simulink model "AUAV_V3_TestSensors"  (R2015a)
settings: Solver=FixedStepDiscrete  StartTime=0.0  StopTime=10.0  FixedStep=T  RelTol=1e-3
PreLoadFcn:
  | %T = 0.0025;
  | MavlinkBus;
  | mcuInit;
  | % Baro Altitude Computation
  | % =========================
  | basePressure = 98192.64;
  | baseTemp = 288.215;
  | lapseRate = -0.00198122;
  | baseHeight = 0;
undefined symbols (not defined in the file): A0, A14, A15, A2, A3, A4, A5, A6, accBiasRateLimit, apSampleTime, B0, bankCommandLimit, barAdjust, baroCutoff, baroCutTemp, baroOffset, baroScale, barTGain1, barTGain2, barTMean1, barTMean2, bda, bde, bdr, bdt, bICda, bICde, bICdr, bICdt, cubeAccelGain16405, cubeGyroGain16405, cubeMagGain16405, D0, D11, D7, D8, daLimit, data, daTrimMax, daTrimMin, deLimit, derivativesConstant, deTrimMax, deTrimMin, drLimit, drTrimMax, drTrimMin, dtLimit, dtTrimMax, dtTrimMin, F2, F3, G0, G13, G15, gaind, GS_location, gyroBiasRateLimit, IC1max, imuOffset_xacc ... (+77)
libraries: MCHP_Blockset x158, simulink x84, SLUGS_Library x31, aerolibconvert2 x6, aerolibutil x4, aerolibtransform2 x3, dspmtrx3 x2, aerolibobsolete x2
(part 8 of 23)

== system AUAV_V3_TestSensors/Trim Vals [updated 4.28.16] ==
  Bufffer IC : Subsystem
  Control Surfaces [dT dA dR dE] : Selector  InputPortWidth=5  Indices=[3 1 4 2]
  Control Surface Input : Subsystem
  "Convert to Microseconds " : Subsystem
  Detect Transition High to Low : Subsystem
  Failsafe : Selector  InputPortWidth=5  Indices=[5]
  Grab I.C. : Subsystem  TreatAsAtomicUnit=on
  Manual or Auto? [navSupport.c] [updated 4.28.16] : MCHP_Blockset/User Functions/C Function Call  ParseFilesChkbx=off  ListFunctions1=Custom Function  Function1=extern uint8_T isApManual(uint16_T u1);  AddHeaderDeclaration=on  Function1Type=when block is updated (default)  FctReturnBlockOut=on  Fct1BlockOut=y1  DataCollected=0  ORDERING=None  SampleTime=-1  MCHP_MASTERLINK=|  PinDigitalInput=[]  PinDigitalOutput=[]  PinAnalogInput=[]
      | AUAV_V3_TestSensors/Microchip Master
      | AUAV V3 Board
      | Busy Flag on D2 (RA6)
  Mean Filter the Transition : Subsystem
  dT Trim : Outport
  dA Trim : Outport  Port=2
  dR Trim : Outport  Port=3
  dE Trim : Outport  Port=4
  Pil Console : Outport  Port=5
  Manual? : Outport  Port=6
  V/I Sensor : Outport  Port=7
  wires:
  Manual or Auto? [navSupport.c] [updated 4.28.16]/1 -> Detect Transition High to Low/1(Switch), Manual?/1
  Control Surface Input/1(Pilot Console) -> Control Surfaces [dT dA dR dE]/1, Failsafe/1
  Control Surfaces [dT dA dR dE]/1 -> Pil Console/1, Bufffer IC/1(Pilot Console)
  Bufffer IC/1(dT_buf) -> Grab I.C./1(dT_buf)
  Bufffer IC/2(dA_buf) -> Grab I.C./2(dA_buf)
  Bufffer IC/3(dR_buf) -> Grab I.C./3(dR_buf)
  Bufffer IC/4(dE_buf) -> Grab I.C./4(dE_buf)
  Grab I.C./4(dE_trim (rad)) -> dE Trim/1
  Grab I.C./3(dR_trim (rad)) -> dR Trim/1
  Grab I.C./2(dA_trim (rad)) -> dA Trim/1
  Grab I.C./1(dT_trim (abs)) -> dT Trim/1
  Detect Transition High to Low/1(Transition) -> Grab I.C./Enable
  Failsafe/1 -> "Convert to Microseconds "/1(IC)
  "Convert to Microseconds "/1(uS) -> Mean Filter the Transition/1(Failsafe)
  Control Surface Input/2(Voltage/Current Sensor) -> V/I Sensor/1
  Mean Filter the Transition/1(filtered) -> Manual or Auto? [navSupport.c] [updated 4.28.16]/1

== system AUAV_V3_TestSensors/Update PWM Commands and Send Telemetry [updated 4.27.16] ==
  PWM(rad) [dT dA dR dE] : Inport
  Pilot Console (IC) [dT dA dR dE] : Inport  Port=2
  Euler_rot : Inport  Port=3
  PQR_rot : Inport  Port=4
  Manual? : Inport  Port=5
  VI : Inport  Port=6
  Convert to Microseconds : Subsystem
  Data Store Read : DataStoreRead  DialogController=Simulink.DDGSource  DataStoreName=SIX_DOF_HIL_FLAG
  Data Store Read1 : DataStoreRead  DataStoreName=X_PLANE_HIL_FLAG
  Demux : Demux
  Demux1 : Demux
  Demux2 : Demux  Outputs=3
  Demux3 : Demux  Outputs=3
  Demux4 : Demux  Outputs=2
  Gain : Gain  Gain=2  OutDataTypeStr=Inherit: Inherit via back propagation
  Generate PWM Signals Based on the Control Type : Subsystem
  Get time3 : DataStoreRead  DataStoreName=time_since_boot_usec  DataStoreElements=time_since_boot_usec
  Output Compare - HW Drive Servo motor : MCHP_Blockset/Pulse Input//Output/Output Compare - HW  Channel="[1     2     3     4]"  Channel_OLD="[1     2     3     4]"  PIN_OC1=Dynamic Options  PIN_OC1_TXT=G0 / P112 / Pin[90]  PIN_OC2=Dynamic Options  PIN_OC2_TXT=E0 / P80 / Pin[93]  PIN_OC3=Dynamic Options  PIN_OC3_TXT=G13 / P125 / Pin[97]  PIN_OC4=Dynamic Options  PIN_OC4_TXT=D7 / P71 / Pin[84]  PIN_OC5=Dynamic Options  PIN_OC5_TXT=D0 / P64 / Pin[72]  PIN_OC6=Dynamic Options  PIN_OC6_TXT=D0 / P64 / Pin[72]  PIN_OC7=Dynamic Options  PIN_OC7_TXT=D0 / P64 / Pin[72]  PIN_OC8=Dynamic Options  PIN_OC8_TXT=D0 / P64 / Pin[72]  PIN_OC9=Dynamic Options  PIN_OC9_TXT=D0 / P64 / Pin[72]  PIN_OC10=Dynamic Options  PIN_OC10_TXT=D0 / P64 / Pin[72]  PIN_OC11=Dynamic Options  PIN_OC11_TXT=D0 / P64 / Pin[72]  PIN_OC12=Dynamic Options  PIN_OC12_TXT=D0 / P64 / Pin[72]  PIN_OC13=Dynamic Options  PIN_OC13_TXT=D0 / P64 / Pin[72]  PIN_OC14=Dynamic Options  PIN_OC14_TXT=D0 / P64 / Pin[72]  PIN_OC15=Dynamic Options  PIN_OC15_TXT=D0 / P64 / Pin[72]  PIN_OC16=Dynamic Options  PIN_OC16_TXT=D0 / P64 / Pin[72]  PIN_OCFA=Dynamic Options  PIN_OCFA_TXT=A0 / P16 / Pin[17]  PIN_OCFB=Dynamic Options  PIN_OCFB_TXT=A0 / P16 / Pin[17]  PIN_OCFC=Dynamic Options  PIN_OCFC_TXT=A0 / P16 / Pin[17]  Channel_UP_Down_Periode="[5     5     5     5]"  PulseTrig=Single pulse triggered by block execution  InputPeriod=are set to the Max time (constant below)  MaxChannel="[0.003   0.003   0.003   0.003]"  MaxChannelUnique=.0001  MaxChannelValue="2.^[ 14.680  14.680  14.680  14.680]  =>  [26249  26249  26249  26249]"  OCxmax="[26249  26249  26249  26249]"  Timer="[1  1  1  1]"  SampleTime=0.02  MCHP_PORT={Output Compare 1}{OC1}7:1:P112;{Output Compare 2}{OC2}7:1:P80;{Output Compare 3}{OC3}7:1:P125;{Output Compare 4}{OC4}7:1:P71;  MCHP_TIMER_REQUEST="{Output Compare 1}{OC1}7:0:1:0:[1  2  3  4  5]:210000;{Output Compare 1}{OC1}7:0:1:0:[1  2  3  4  5]:210000;{Output Compare 1}{OC1}7:0:1:0:[1  2  3  4  5]:210000;{Output Compare 1}{OC1}7:0:1:0:[1  2  3  4  5]:210000;"  MCHP_TIMER_RESULT=[1 26249.000000000011 ;1 26249.000000000011 ;1 26249.000000000011 ;1 26249.000000000011 ]  MCHP_MASTERLINK=|
      | AUAV_V3_TestSensors/Microchip Master
      | AUAV V3 Board
      | Busy Flag on D2 (RA6)
  PWM High Speed : MCHP_Blockset/PWM IO/PWM High Speed  Commented=on  pop1=[1]  chk1="[1  1  1  0]"  chkHL1="[1  1  1  1  0  0  1 ; 1  1  1  1  0  0  1]"  maxP1="[0.001       0.001       0.001       0.001       0.001       0.001       0.001 ; 0.001       0.001      1e-006       0.001       0.001       0.001       0.001]"  InitP2="[0.001       0.001       0.001       0.001       0.001       0.001       0.001 ; 0.001       0.001       0.001       0.001       0.001       0.001       0.001]"  chkP2="[0  0  0  0  1  1  1 ; 1  0  0  1  1  1  1]"  InitDC="[0.0005       0.0004       0.0003        0.001        0.001        0.001           50 ; 0.001        0.001        0.001        0.001        0.001        0.001           50]"  chkDC="[1  1  1  1  1  1  1 ; 0  0  0  1  1  1  1]"  InitPh="[0           0           0       0.001       0.001       0.001       0.001 ; 0           0           0       0.001       0.001       0.001       0.001]"  chkPh="[0  0  0  1  1  1  1 ; 0  0  0  1  1  1  1]"  edSEvTrigx={'0.0006','-1','-1','-1','-1','-1','-1'}  chkSEvTrigx="[0  0  0  0  1  1  1]"  popFlt="[1  1  1  1  1  1  1]"  popFltPin="[48  48  48  48  48  48  48]"  popFltPinRp="[1  1  1  1  1  1  1]"  popFltActivH="[1  2  1  1  1  1  1]"  popFltForceH="[2  2  2  2  2  2  2]"  popFltForceL="[1  1  1  1  1  1  1]"  chkFltBlkOut="[0  0  0  0  0  0  0]"  popDT="[3  3  3  3  3  3  3]"  edDTRx="[0.02      1e-005       0.001      1e-005      1e-005      1e-005      1e-005]"  edAltDTRx="[1e-005      0.0001      1e-005      1e-005      1e-005      1e-005      1e-005]"  S_INPUT="[5  5  5  5]"  S_INPUT_Size=[1 1 1 1]  S_OUTPUT=[]  S_OUTPUT_Size=[]  S_DWORK_Type=[]  S_DWORK_Size=[]  ADC_VARTRIG={PWM Primary Special Event Trigger;6}  SampleTime=-1  ORDERING=None  MCHP_PORT={PWM1H}{PWM1H}4:4:E1;{PWM1L}{PWM1L}4:4:E0;{PWM2H}{PWM2H}4:4:E3;{PWM2L}{PWM2L}4:4:E2;{PWM3H}{PWM3H}4:4:E5;{PWM3L}{PWM3L}4:4:E4;{PWM4H}{PWM4H}4:4:E7;{PWM4L}{PWM4L}4:4:E6;  MCHP_MASTERLINK=|  MCHP_VERSION=v3.38
      | AUAV_V3_TestSensors/Microchip Master
      | AUAV V3 Board
      | Busy Flag on D2 (RA6)
  Rate Transition : RateTransition
  Send_Cmd_6DOF_HIL : Subsystem
  Send_Cmd_X_Plane_HIL : Subsystem
  "[ dA dE dT dR ]" : Selector  InputPortWidth=4  Indices=[2 4 1 3]
  mlAttitude : DataStoreWrite  DataStoreName=mlVISensor  DataStoreElements=mlVISensor.voltage#mlVISensor.reading2
  mlAttitudeEuler : DataStoreWrite  DialogController=Simulink.DDGSource  DataStoreName=mlAttitudeSol  DataStoreElements=mlAttitudeSol.roll#mlAttitudeSol.pitch#mlAttitudeSol.yaw#mlAttitudeSol.time_boot_ms
  mlAttitudePQR : DataStoreWrite  DialogController=Simulink.DDGSource  DataStoreName=mlAttitudeSol  DataStoreElements=mlAttitudeSol.rollspeed#mlAttitudeSol.pitchspeed#mlAttitudeSol.yawspeed
  mlHeartbeatLocal : DataStoreRead  DataStoreName=mlHeartbeatLocal  DataStoreElements=mlHeartbeatLocal.custom_mode
  mlPwmCommands : DataStoreWrite  DialogController=Simulink.DDGSource  DataStoreName=mlPwmCommands  DataStoreElements=mlPwmCommands.servo1_raw#mlPwmCommands.servo2_raw#mlPwmCommands.servo3_raw#mlPwmCommands.servo4_raw#mlPwmCommands.time_usec
  wires:
  Generate PWM Signals Based on the Control Type/1(PWM) -> "[ dA dE dT dR ]"/1, Convert to Microseconds/1(PWM)  "[dT dA dR dE]"
  PWM(rad) [dT dA dR dE]/1 -> Generate PWM Signals Based on the Control Type/1(PWM(rad))
  Pilot Console (IC) [dT dA dR dE]/1 -> Generate PWM Signals Based on the Control Type/2(Pilot Console (IC))
  Manual?/1 -> Generate PWM Signals Based on the Control Type/3(isManual?)
  mlHeartbeatLocal/1 -> Generate PWM Signals Based on the Control Type/4(Nav Mode)
  Convert to Microseconds/1(uS) -> Demux1/1
  Demux1/1 -> mlPwmCommands/1
  Demux1/2 -> mlPwmCommands/2
  Demux1/3 -> mlPwmCommands/3
  Demux1/4 -> mlPwmCommands/4
  Demux2/1 -> mlAttitudeEuler/1
  Demux2/2 -> mlAttitudeEuler/2
  Demux2/3 -> mlAttitudeEuler/3
  Euler_rot/1 -> Demux2/1
  Demux3/1 -> mlAttitudePQR/1
  Demux3/2 -> mlAttitudePQR/2
  Demux3/3 -> mlAttitudePQR/3
  PQR_rot/1 -> Demux3/1
  Demux4/1 -> mlAttitude/1
  Demux4/2 -> mlAttitude/2
  VI/1 -> Demux4/1
  Demux/1 -> Output Compare - HW Drive Servo motor/1
  Demux/2 -> Output Compare - HW Drive Servo motor/2
  Demux/3 -> Output Compare - HW Drive Servo motor/3
  Demux/4 -> Output Compare - HW Drive Servo motor/4
  Get time3/1 -> mlPwmCommands/5, mlAttitudeEuler/4
  Data Store Read/1 -> Send_Cmd_6DOF_HIL/Enable
  Data Store Read1/1 -> Send_Cmd_X_Plane_HIL/Enable
  "[ dA dE dT dR ]"/1 -> Rate Transition/1
  Rate Transition/1 -> Gain/1
  Gain/1 -> Demux/1

== system AUAV_V3_TestSensors/get Nav Vars [updated 4.28.16] ==
  Attitude : Inport
  Accel : Inport  Port=2
  Accel. Bias : Inport  Port=3
  Angle Conversion : aerolibconvert2/Angle Conversion  IU=deg  OU=rad
  Demux : Demux  Outputs=3
  Direction Cosine Matrix to Rotation Angles : aerolibtransform2/Direction Cosine Matrix to Rotation Angles  rotationOrder=ZYX  lim=Default
      settings: AttributesFormatString=Rotation Order: %<rotationOrder>
  Embedded MATLAB Function1 : MATLAB Function  TreatAsAtomicUnit=on
  Euler : Selector  InputPortWidth=6  Indices=[1 2 3]
  Euler Angles to Direction Cosine Matrix1 : aerolibobsolete/Euler Angles to  Direction Cosine Matrix
  Euler Angles to Direction Cosine Matrix2 : aerolibobsolete/Euler Angles to  Direction Cosine Matrix
  Math Function : Math  Operator=transpose  SaturateOnIntegerOverflow=on
  Mux : Mux  Inputs=3
  PAR_CONFIG_ROLL_R PAR_CONFIG_PITCH_R PAR_CONFIG_YAW_R : DataStoreRead  DialogController=Simulink.DDGSource  DataStoreName=mlParamInterface  DataStoreElements=mlParamInterface.param(16)#mlParamInterface.param(17)#mlParamInterface.param(18)
  Product{,1..3} (4 alike) : Product  Multiplication=Matrix(*)  RndMeth=Zero
  Rates : Selector  InputPortWidth=6  Indices=[4 5 6]
  Selector : Selector  InputPortWidth=6  Indices=[1 2 5 6]
  Selector1 : Selector  InputPortWidth=3  Indices=[2]
  Sum : Sum  Inputs=+|+
  myMux Fun1 : MATLAB Function  TreatAsAtomicUnit=on
  myMux Fun2 : MATLAB Function  TreatAsAtomicUnit=on
  "[phi the q r]" : Outport
  Euler Rot : Outport  Port=2
  PQR Rot : Outport  Port=3
  Yb Accel : Outport  Port=4
  wires:
  Selector/1 -> "[phi the q r]"/1
  Euler/1 -> Euler Angles to Direction Cosine Matrix2/1
  Euler Angles to Direction Cosine Matrix2/1 -> Product/2
  Euler Angles to Direction Cosine Matrix1/1 -> Math Function/1
  Angle Conversion/1 -> Euler Angles to Direction Cosine Matrix1/1
  Product/1 -> Direction Cosine Matrix to Rotation Angles/1
  Rates/1 -> Product1/2
  myMux Fun1/1(y) -> Euler Rot/1, myMux Fun2/1(u1)
  Product1/1 -> myMux Fun2/2(u2), PQR Rot/1
  myMux Fun2/1(y) -> Selector/1
  Math Function/1 -> Product/1, Product1/1, Product2/1, Product3/1
  Accel/1 -> Product2/2
  Accel. Bias/1 -> Product3/2
  Product2/1 -> Sum/1
  Product3/1 -> Sum/2
  Sum/1 -> Selector1/1
  Selector1/1 -> Yb Accel/1
  Demux/1 -> Embedded MATLAB Function1/1(u)
  Direction Cosine Matrix to Rotation Angles/1 -> Demux/1
  Demux/2 -> myMux Fun1/2(u2)
  Demux/3 -> myMux Fun1/1(u1)
  Embedded MATLAB Function1/1(y) -> myMux Fun1/3(u3)
  Attitude/1 -> Euler/1, Rates/1
  PAR_CONFIG_ROLL_R PAR_CONFIG_PITCH_R PAR_CONFIG_YAW_R/2 -> Mux/2
  PAR_CONFIG_ROLL_R PAR_CONFIG_PITCH_R PAR_CONFIG_YAW_R/1 -> Mux/1
  PAR_CONFIG_ROLL_R PAR_CONFIG_PITCH_R PAR_CONFIG_YAW_R/3 -> Mux/3
  Mux/1 -> Angle Conversion/1

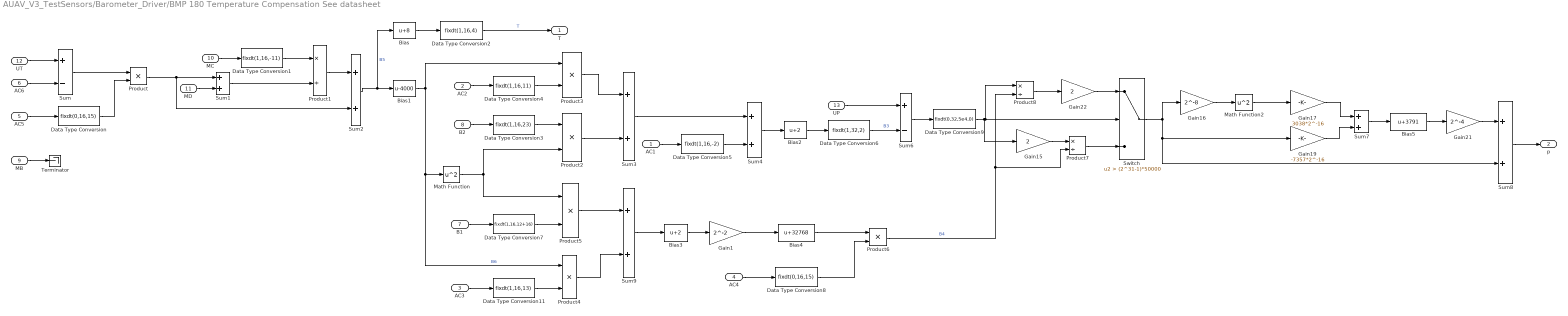
== system AUAV_V3_TestSensors/Barometer_Driver/BMP 180 Temperature Compensation See datasheet ==
  AC1 : Inport
  AC2 : Inport  Port=2
  AC3 : Inport  Port=3
  AC4 : Inport  Port=4
  AC5 : Inport  Port=5
  AC6 : Inport  Port=6
  B1 : Inport  Port=7
  B2 : Inport  Port=8
  MB : Inport  Port=9
  MC : Inport  Port=10
  MD : Inport  Port=11
  UT : Inport  Port=12
  UP : Inport  Port=13
  Bias : Bias  Bias=8
  Bias1 : Bias  Bias=-4000
  Bias2 : Bias  Bias=2
  Bias3 : Bias  Bias=2
  Bias4 : Bias  Bias=32768
  Bias5 : Bias  Bias=3791
  Data Type Conversion : DataTypeConversion  OutDataTypeStr=fixdt(0,16,15)  ConvertRealWorld=Stored Integer (SI)
  Data Type Conversion1 : DataTypeConversion  OutDataTypeStr=fixdt(1,16,-11)  ConvertRealWorld=Stored Integer (SI)
  Data Type Conversion11 : DataTypeConversion  OutDataTypeStr=fixdt(1,16,13)  ConvertRealWorld=Stored Integer (SI)
  Data Type Conversion2 : DataTypeConversion  OutDataTypeStr=fixdt(1,16,4)  ConvertRealWorld=Stored Integer (SI)
  Data Type Conversion3 : DataTypeConversion  OutDataTypeStr=fixdt(1,16,23)  ConvertRealWorld=Stored Integer (SI)
  Data Type Conversion4 : DataTypeConversion  OutDataTypeStr=fixdt(1,16,11)  ConvertRealWorld=Stored Integer (SI)
  Data Type Conversion5 : DataTypeConversion  OutDataTypeStr=fixdt(1,16,-2)  ConvertRealWorld=Stored Integer (SI)
  Data Type Conversion6 : DataTypeConversion  OutDataTypeStr=fixdt(1,32,2)  ConvertRealWorld=Stored Integer (SI)
  Data Type Conversion7 : DataTypeConversion  OutDataTypeStr=fixdt(1,16,12+16)  ConvertRealWorld=Stored Integer (SI)
  Data Type Conversion8 : DataTypeConversion  OutDataTypeStr=fixdt(0,16,15)  ConvertRealWorld=Stored Integer (SI)
  Data Type Conversion9 : DataTypeConversion  OutDataTypeStr=fixdt(0,32,5e4,0)  ConvertRealWorld=Stored Integer (SI)
  Gain1 : Gain  Gain=2^-2  OutDataTypeStr=int32
  Gain15 : Gain  Gain=2  OutDataTypeStr=uint32  RndMeth=Round
  Gain16 : Gain  Gain=2^-8  OutDataTypeStr=int32  RndMeth=Round
  Gain17 : Gain  Gain=3038*2^-16  OutDataTypeStr=uint32
  Gain19 : Gain  Gain=-7357*2^-16  ParamDataTypeStr=fixdt(1,16)  OutDataTypeStr=int32
  Gain21 : Gain  Gain=2^-4  OutDataTypeStr=Inherit: Same as input
  Gain22 : Gain  Gain=2  OutDataTypeStr=Inherit: Same as input
  Math Function : Math  Operator=square  SaturateOnIntegerOverflow=on  OutDataTypeStr=Inherit: Inherit via internal rule
  Math Function2 : Math  Operator=square  OutDataTypeStr=uint32  SaturateOnIntegerOverflow=on
  Product : Product  RndMeth=Round  OutDataTypeStr=Inherit: Same as first input
  Product1 : Product  Inputs=*/  OutDataTypeStr=int16  RndMeth=Round
  Product2 : Product  OutDataTypeStr=int16
  Product3 : Product  OutDataTypeStr=Inherit: Same as first input
  Product4 : Product  OutDataTypeStr=int16
  Product5 : Product  OutDataTypeStr=int16
  Product6 : Product  OutDataTypeStr=uint32
  Product7 : Product  Inputs=*/  RndMeth=Round
  Product8 : Product  Inputs=*/  OutDataTypeStr=uint32  RndMeth=Round
  Sum : Sum  Inputs=+-  RndMeth=Round
  Sum1 : Sum  RndMeth=Round  OutDataTypeStr=Inherit: Same as first input
  Sum2 : Sum  AccumDataTypeStr=int16  OutDataTypeStr=int16  RndMeth=Round
  Sum3 : Sum
  Sum4 : Sum  OutDataTypeStr=int32
  Sum6 : Sum  Inputs=+-  AccumDataTypeStr=uint32  OutDataTypeStr=uint32
  Sum7 : Sum  AccumDataTypeStr=int32  OutDataTypeStr=int32
  Sum8 : Sum  AccumDataTypeStr=int32  OutDataTypeStr=Inherit: Same as accumulator  RndMeth=Round
  Sum9 : Sum
  Switch : Switch  Criteria=u2 > Threshold  Threshold=(2^31-1)*50000
  Terminator : Terminator
  T : Outport
  p : Outport  Port=2
  wires:
  MB/1 -> Terminator/1
  Sum9/1 -> Bias3/1
  Product4/1 -> Sum9/2
  Product5/1 -> Sum9/1
  Product2/1 -> Sum3/2
  Product3/1 -> Sum3/1
  Data Type Conversion3/1 -> Product2/1
  Data Type Conversion11/1 -> Product4/2
  Product1/1 -> Sum2/1
  Data Type Conversion8/1 -> Product6/2
  Data Type Conversion7/1 -> Product5/2
  Data Type Conversion4/1 -> Product3/2
  Math Function/1 -> Product5/1, Product2/2
  Data Type Conversion/1 -> Product/2
  Bias5/1 -> Gain21/1
  Sum8/1 -> p/1
  Gain21/1 -> Sum8/1
  Sum7/1 -> Bias5/1
  Gain17/1 -> Sum7/1
  Gain19/1 -> Sum7/2
  Math Function2/1 -> Gain17/1
  Gain16/1 -> Math Function2/1
  Switch/1 -> Gain19/1, Sum8/2, Gain16/1
  Product7/1 -> Switch/3
  Product8/1 -> Gain22/1
  Data Type Conversion9/1 -> Gain15/1, Product8/1, Switch/2
  Sum6/1 -> Data Type Conversion9/1
  UP/1 -> Sum6/1
  Data Type Conversion6/1 -> Sum6/2  "B3"
  Product6/1 -> Product8/2, Product7/2  "B4"
  Bias4/1 -> Product6/1
  AC4/1 -> Data Type Conversion8/1
  Gain1/1 -> Bias4/1
  Bias3/1 -> Gain1/1
  B1/1 -> Data Type Conversion7/1
  AC3/1 -> Data Type Conversion11/1
  Sum4/1 -> Bias2/1
  Data Type Conversion5/1 -> Sum4/2
  Bias2/1 -> Data Type Conversion6/1
  AC1/1 -> Data Type Conversion5/1
  Sum3/1 -> Sum4/1
  AC2/1 -> Data Type Conversion4/1
  B2/1 -> Data Type Conversion3/1
  Bias1/1 -> Product3/1, Product4/1, Math Function/1  "B6"
  MC/1 -> Data Type Conversion1/1
  Data Type Conversion2/1 -> T/1  "T"
  Bias/1 -> Data Type Conversion2/1
  Sum1/1 -> Product1/2
  Sum2/1 -> Bias1/1, Bias/1  "B5"
  Product/1 -> Sum1/1, Sum2/2
  MD/1 -> Sum1/2
  AC5/1 -> Data Type Conversion/1
  Sum/1 -> Product/1
  AC6/1 -> Sum/2
  UT/1 -> Sum/1
  Data Type Conversion1/1 -> Product1/1
  Gain22/1 -> Switch/1
  Gain15/1 -> Product7/1

== system AUAV_V3_TestSensors/Barometer_Driver/Baro Altimeter ==
  Static (Pa) : Inport
  Compute Barometric Height : Subsystem  mask{baseTemp=baseTemp, LapseRate=lapseRate}
      mask prompts: baseTemp "Base Station Temperature (K)"; LapseRate "Lapse Rate (C/ft)"
      mask help:
      | Produces Altitude in meters from Barometric Pressure in Pascals. Altitude is valid from MSL to 6000 ft.
      |
      | The method implemented here was developed by Ren Curry
  Constant5 : Constant  Value=baseHeight  OutDataTypeStr=single
  Enabled Subsystem : Subsystem  TreatAsAtomicUnit=on
  Enables/Disables the Computation of initial Baro Bias : MATLAB Function  TreatAsAtomicUnit=on
  Initial Baro Bias : Subsystem  TreatAsAtomicUnit=on
  Logical Operator : Logic  Operator=NOT  AllPortsSameDT=off  OutDataTypeStr=boolean
  Sum1 : Sum  Inputs=++|  OutDataTypeStr=single
  Zero Out Height : Subsystem  TreatAsAtomicUnit=on
  Altitude : Outport
  wires:
  Enabled Subsystem/1(Out1) -> Altitude/1
  Sum1/1 -> Enabled Subsystem/1(In1)
  Logical Operator/1 -> Enabled Subsystem/Enable
  Zero Out Height/1(Height Offset) -> Sum1/1
  Initial Baro Bias/1(Baro (Gnd)) -> Compute Barometric Height/2(Base Pressure (Pa))
  Constant5/1 -> Zero Out Height/1(Base Height), Compute Barometric Height/1(Base Height (m))
  Enables/Disables the Computation of initial Baro Bias/1(tOut) -> Logical Operator/1, Zero Out Height/Enable, Initial Baro Bias/Enable
  Static (Pa)/1 -> Compute Barometric Height/3(Baro (Pa)), Initial Baro Bias/1(Baro (Pa))
  Compute Barometric Height/1("Altitude, m") -> Sum1/2, Zero Out Height/2(Computed Height)

== system AUAV_V3_TestSensors/Barometer_Driver/Disable path through in HIL Subsystem ==
  In1 : Inport
  In2 : Inport  Port=2
  Enable : EnablePort
  Update RawPressure : DataStoreWrite  DataStoreName=mlRawPressureData  DataStoreElements=mlRawPressureData.press_abs#mlRawPressureData.temperature
  wires:
  In1/1 -> Update RawPressure/1
  In2/1 -> Update RawPressure/2

== system AUAV_V3_TestSensors/Barometer_Driver/Disable path through in HIL Subsystem1 ==
  In1 : Inport
  In2 : Inport  Port=2
  Enable : EnablePort
  Update ScaledPressure : DataStoreWrite  DialogController=Simulink.DDGSource  DataStoreName=mlAirData  DataStoreElements=mlAirData.temperature#mlAirData.press_abs
  wires:
  In1/1 -> Update ScaledPressure/1
  In2/1 -> Update ScaledPressure/2

== system AUAV_V3_TestSensors/Barometer_Driver/I2C Initialisation Read EEPROM Calibration data Once (Blocking Function) ==
  Enable : EnablePort
  BUS I2C Initialize BMP180 read Calibration data @ 100Hz : MCHP_Blockset/BUS I2C/BUS I2C MASTER  I2CRef=2  I2C_IntPriority=6  I2Csequence_txt="Initial-Configuration$     ---     $Start$Write Address:{[0x77]}    % BMP180 Address$Write Data (x1)  Write:{[0xAA ]}  $Re-Start    % Re-Start when not followed with either Read or Write action rethrow Address$Read Data (x22)  Read:{Out 9}$Stop"  I2Csequence_num=[BFF0000000000000 40E0600000000000 40F86A0000000000 410065D9C7810E65]$[4070000000000000]$[3FF0000000000000 40E0200000000000 40F86A0000000000 40F866E066594CA2]$[4040000000000000 0000000000000000 0000000000000000 405DC00000000000]$[4050000000000000 3FF0000000000000 0000000000000000 4065400000000000]$[4008000000000000 40E0000000000000 40F86A0000000000 410065D9C7810E65]$[4060000000000000 4036000000000000]$[4000000000000000 40E0600000000000 40F86A0000000000 410065D9C7810E65]  InitialConfigurationNum=0  PIN_SDA_TXT=A3 / Pin[59]  PIN_SCL_TXT=A2 / Pin[58]  S_INPUT="[5  5]"  S_OUTPUT=[5]  S_INPUT_Size="[2  2]"  S_OUTPUT_Size=[4]  BlockingMode=on  SampleTime=.01  MCHP_MASTERLINK=|  MCHP_PORT={I2C 2 Clock}{SCL2}13:0:A2;{I2C 2 SDA}{SDA2}13:0:A3;  ORDERING=0
      | AUAV_V3_TestSensors/Microchip Master
      | AUAV V3 Board
      | Busy Flag on D2 (RA6)
  Data Type Conversion{1..8} (8 alike) : DataTypeConversion  OutDataTypeStr=int16  ConvertRealWorld=Stored Integer (SI)
  Data Type Conversion10 : DataTypeConversion  OutDataTypeStr=uint16  ConvertRealWorld=Stored Integer (SI)  LockScale=on
  Data Type Conversion11 : DataTypeConversion  OutDataTypeStr=uint16  ConvertRealWorld=Stored Integer (SI)  LockScale=on
  Data Type Conversion9 : DataTypeConversion  OutDataTypeStr=uint16  ConvertRealWorld=Stored Integer (SI)  LockScale=on
  Demux4 : Demux  Outputs=22
  Pack10 : Subsystem
  Pack11 : Subsystem
  Pack12 : Subsystem
  Pack2 : Subsystem
  Pack3 : Subsystem
  Pack4 : Subsystem
  Pack5 : Subsystem
  Pack6 : Subsystem
  Pack7 : Subsystem
  Pack8 : Subsystem
  Pack9 : Subsystem
  Rate Transition{2..12} (11 alike) : RateTransition  Deterministic=off
  Out1 : Outport
  Out2 : Outport  Port=2
  Out3 : Outport  Port=3
  Out4 : Outport  Port=4
  Out5 : Outport  Port=5
  Out6 : Outport  Port=6
  Out7 : Outport  Port=7
  Out8 : Outport  Port=8
  Out9 : Outport  Port=9
  Out10 : Outport  Port=10
  Out11 : Outport  Port=11
  wires:
  BUS I2C Initialize BMP180 read Calibration data @ 100Hz/1 -> Demux4/1
  Demux4/12 -> Pack7/2(Low)
  Data Type Conversion10/1 -> Rate Transition6/1  "U3 CH5"
  Data Type Conversion1/1 -> Rate Transition3/1  "U3 CH2"
  Data Type Conversion2/1 -> Rate Transition2/1  "U3 CH1"
  Data Type Conversion11/1 -> Rate Transition7/1  "U3 CH6"
  Data Type Conversion5/1 -> Rate Transition9/1  "U3 CH8"
  Data Type Conversion8/1 -> Rate Transition12/1  "U3 CH11"
  Data Type Conversion6/1 -> Rate Transition10/1  "U3 CH9"
  Data Type Conversion4/1 -> Rate Transition8/1  "U3 CH7"
  Data Type Conversion3/1 -> Rate Transition4/1  "U3 CH3"
  Data Type Conversion7/1 -> Rate Transition11/1  "U3 CH10"
  Data Type Conversion9/1 -> Rate Transition5/1  "U3 CH4"
  Pack6/1(Out1) -> Data Type Conversion10/1
  Pack5/1(Out1) -> Data Type Conversion9/1
  Pack7/1(Out1) -> Data Type Conversion11/1
  Pack8/1(Out1) -> Data Type Conversion4/1
  Pack9/1(Out1) -> Data Type Conversion5/1
  Pack10/1(Out1) -> Data Type Conversion6/1
  Pack11/1(Out1) -> Data Type Conversion7/1
  Pack12/1(Out1) -> Data Type Conversion8/1
  Pack4/1(Out1) -> Data Type Conversion3/1
  Demux4/15 -> Pack9/1(Hi)
  Pack3/1(Out1) -> Data Type Conversion1/1
  Pack2/1(Out1) -> Data Type Conversion2/1
  Demux4/22 -> Pack12/2(Low)
  Demux4/14 -> Pack8/2(Low)
  Demux4/16 -> Pack9/2(Low)
  Demux4/17 -> Pack10/1(Hi)
  Demux4/18 -> Pack10/2(Low)
  Demux4/19 -> Pack11/1(Hi)
  Demux4/20 -> Pack11/2(Low)
  Demux4/21 -> Pack12/1(Hi)
  Demux4/2 -> Pack2/2(Low)
  Demux4/13 -> Pack8/1(Hi)
  Demux4/11 -> Pack7/1(Hi)
  Demux4/9 -> Pack6/1(Hi)
  Demux4/10 -> Pack6/2(Low)
  Demux4/1 -> Pack2/1(Hi)
  Demux4/3 -> Pack3/1(Hi)
  Demux4/4 -> Pack3/2(Low)
  Demux4/6 -> Pack4/2(Low)
  Demux4/5 -> Pack4/1(Hi)
  Demux4/7 -> Pack5/1(Hi)
  Demux4/8 -> Pack5/2(Low)
  Rate Transition12/1 -> Out11/1
  Rate Transition10/1 -> Out9/1
  Rate Transition11/1 -> Out10/1
  Rate Transition9/1 -> Out8/1
  Rate Transition3/1 -> Out2/1
  Rate Transition7/1 -> Out6/1
  Rate Transition4/1 -> Out3/1
  Rate Transition6/1 -> Out5/1
  Rate Transition8/1 -> Out7/1
  Rate Transition2/1 -> Out1/1
  Rate Transition5/1 -> Out4/1

== system AUAV_V3_TestSensors/Barometer_Driver/LPF 1Hz ==
  Input : Inport
  Delay11 : Delay  DelayLength=1  InitialCondition=0  InputProcessing=Inherited
  SumA21 : Sum  Inputs=|++  AccumDataTypeStr=fixdt(0,32,15)  OutDataTypeStr=Inherit: Same as accumulator  SaturateOnIntegerOverflow=on
  SumB21 : Sum  Inputs=|++  AccumDataTypeStr=fixdt(0,32,16)  OutDataTypeStr=uint16  SaturateOnIntegerOverflow=on
  a(2)(1) : Gain  Gain=0.9390625058174924  ParamDataTypeStr=fixdt(0,16,16)  OutDataTypeStr=fixdt(0,32,15)  SaturateOnIntegerOverflow=on
  s(1) : Gain  Gain=0.030468747091253828  ParamDataTypeStr=fixdt(0,16,20)  OutDataTypeStr=fixdt(0,32,16)  SaturateOnIntegerOverflow=on
  Output : Outport
  wires:
  s(1)/1 -> SumA21/1
  SumA21/1 -> SumB21/1, Delay11/1
  a(2)(1)/1 -> SumA21/2
  Delay11/1 -> SumB21/2, a(2)(1)/1
  SumB21/1 -> Output/1
  Input/1 -> s(1)/1

== system AUAV_V3_TestSensors/Barometer_Driver/LPF 1Hz1 ==
  Input : Inport
  Delay11 : Delay  DelayLength=1  InitialCondition=0  InputProcessing=Inherited
  SumA21 : Sum  Inputs=|++  AccumDataTypeStr=fixdt(0,32,15)  OutDataTypeStr=Inherit: Same as accumulator  SaturateOnIntegerOverflow=on
  SumB21 : Sum  Inputs=|++  AccumDataTypeStr=fixdt(0,32,16)  OutDataTypeStr=uint16  SaturateOnIntegerOverflow=on
  a(2)(1) : Gain  Gain=0.9390625058174924  ParamDataTypeStr=fixdt(0,16,16)  OutDataTypeStr=fixdt(0,32,15)  SaturateOnIntegerOverflow=on
  s(1) : Gain  Gain=0.030468747091253828  ParamDataTypeStr=fixdt(0,16,20)  OutDataTypeStr=fixdt(0,32,16)  SaturateOnIntegerOverflow=on
  Output : Outport
  wires:
  Input/1 -> s(1)/1
  SumB21/1 -> Output/1
  Delay11/1 -> a(2)(1)/1, SumB21/2
  a(2)(1)/1 -> SumA21/2
  SumA21/1 -> Delay11/1, SumB21/1
  s(1)/1 -> SumA21/1

== system AUAV_V3_TestSensors/Barometer_Driver/Pack ==
  Hi : Inport
  Low : Inport  Port=2
  Bitwise Operator : simulink/Logic and Bit Operations/Bitwise Operator  logicop=OR  UseBitMask=off  NumInputPorts=2  BitMask=bin2dec('11011001')  BitMaskRealWorld=Stored Integer
  Data Type Conversion1 : DataTypeConversion  OutDataTypeStr=uint16  ConvertRealWorld=Stored Integer (SI)
  Data Type Conversion2 : DataTypeConversion  OutDataTypeStr=uint16  ConvertRealWorld=Stored Integer (SI)
  Data Type Conversion3 : DataTypeConversion  OutDataTypeStr=uint16  ConvertRealWorld=Stored Integer (SI)
  Gain : Gain  Gain=2^8  OutDataTypeStr=Inherit: Same as input
  Out1 : Outport
  wires:
  Data Type Conversion3/1 -> Bitwise Operator/2
  Low/1 -> Data Type Conversion3/1
  Data Type Conversion1/1 -> Gain/1
  Bitwise Operator/1 -> Data Type Conversion2/1
  Hi/1 -> Data Type Conversion1/1
  Gain/1 -> Bitwise Operator/1
  Data Type Conversion2/1 -> Out1/1

== system AUAV_V3_TestSensors/Barometer_Driver/Pack1 ==
  Hi : Inport
  Low : Inport  Port=2
  Bitwise Operator : simulink/Logic and Bit Operations/Bitwise Operator  logicop=OR  UseBitMask=off  NumInputPorts=2  BitMask=bin2dec('11011001')  BitMaskRealWorld=Stored Integer
  Data Type Conversion1 : DataTypeConversion  OutDataTypeStr=uint16  ConvertRealWorld=Stored Integer (SI)
  Data Type Conversion2 : DataTypeConversion  OutDataTypeStr=uint16  ConvertRealWorld=Stored Integer (SI)
  Data Type Conversion3 : DataTypeConversion  OutDataTypeStr=uint16  ConvertRealWorld=Stored Integer (SI)
  Gain : Gain  Gain=2^8  OutDataTypeStr=Inherit: Same as input
  Out1 : Outport
  wires:
  Gain/1 -> Bitwise Operator/1
  Hi/1 -> Data Type Conversion1/1
  Bitwise Operator/1 -> Data Type Conversion2/1
  Data Type Conversion1/1 -> Gain/1
  Low/1 -> Data Type Conversion3/1
  Data Type Conversion3/1 -> Bitwise Operator/2
  Data Type Conversion2/1 -> Out1/1

== system AUAV_V3_TestSensors/Control Surface Input/PilotConsole ==
  In1 : Inport
  In2 : Inport  Port=2
  In3 : Inport  Port=3
  In4 : Inport  Port=4
  In5 : Inport  Port=5
  Control Surfaces [dT dA dR dE Failsafe] : Selector  InputPortWidth=5  Indices=[1 2 3 4 5]
  "Convert to Microseconds " : Subsystem
  Demux : Demux  Outputs=5
  Update Control Surface DATA : DataStoreWrite  DialogController=Simulink.DDGSource  DataStoreName=mlPilotConsoleData  DataStoreElements=mlRC_Commands.chan1_raw#mlRC_Commands.chan2_raw#mlRC_Commands.chan3_raw#mlRC_Commands.chan4_raw#mlRC_Commands.chan5_raw
  myMux Fun5 : MATLAB Function  TreatAsAtomicUnit=on
  Pilot Console : Outport
  wires:
  In5/1 -> myMux Fun5/5(u5)
  In1/1 -> myMux Fun5/1(u1)
  In3/1 -> myMux Fun5/3(u3)
  In4/1 -> myMux Fun5/4(u4)
  Demux/1 -> Update Control Surface DATA/1
  Demux/4 -> Update Control Surface DATA/4
  In2/1 -> myMux Fun5/2(u2)
  Demux/5 -> Update Control Surface DATA/5
  "Convert to Microseconds "/1(uS) -> Control Surfaces [dT dA dR dE Failsafe]/1
  Demux/2 -> Update Control Surface DATA/2
  Demux/3 -> Update Control Surface DATA/3
  Control Surfaces [dT dA dR dE Failsafe]/1 -> Pilot Console/1, Demux/1
  myMux Fun5/1(y) -> "Convert to Microseconds "/1(IC)

== system AUAV_V3_TestSensors/IMU_Mag_Driver/BUS SPI Read MPU 6050 ==
  "BUS SPI Read MPU 6050 Axyz, T°, Gxyz (100 Hz)" : MCHP_Blockset/BUS SPI/BUS SPI  SPIRef=1  DMA="[0  2  3]"  SPI_IntPriority=5  SPIsequence_txt="Initial-Configuration$     ---     $Set Port E4 / Pin[100] to 0    % /CS$Write only (x1)  Write:{[0xBA00]}      % read one byte before$Read only (x3)  Read:{Axyz}    % Accelerometers$Read only (x1)  Read:{T°}    % Temperature$Read only (x3)  Read:{Gxyz}    % rate gyros$Set Port E4 / Pin[100] to 1    % /CS"  SPIsequence_num=[BFF0000000000000 4091D00000000000 0000000000000000 40E0000000000000 4116409C00000000 4116409D55555555]$[4070000000000000]$[4010000000000000 4051000000000000 0000000000000000]$[3FF0000000000000 3FF0000000000000 0000000000000000 40E7400000000000]$[4000000000000000 4008000000000000]$[4000000000000000 3FF0000000000000]$[4000000000000000 4008000000000000]$[4010000000000000 4051000000000000 3FF0000000000000]  PIN_SDI_TXT=E3 / P83 / Pin[99]  PIN_SDO_TXT=E2 / P82 / Pin[98]  PIN_SCK_TXT=G15 / P127 / Pin[1]  PIN_SS_TXT=B0 / Pin[21]  S_INPUT="[5  5]"  S_OUTPUT=[5]  S_INPUT_Size="[2  2]"  S_OUTPUT_Size=[4]  BlockingMode=off  SampleTime=[.01]  MCHP_MASTERLINK=|  MCHP_PORT={SPI 1 input}{SDI1}12:0:P83;{SPI 1 output}{SDO1}12:1:P82;{SPI 1 Clock output}{SCK1}12:1:P127;{SPI 1 Digital output}{SPI1-DOU}12:1:E4;{SPI 1 Digital output}{SPI1-DOU}12:1:E4;  ORDERING=0
      | AUAV_V3_TestSensors/Microchip Master
      | AUAV V3 Board
      | Busy Flag on D2 (RA6)
  Bias : Bias  Bias=-468
  Bias1 : Bias  Bias=-178
  Bias10 : Bias  Bias=imuOffset_ygyro
  Bias11 : Bias  Bias=imuOffset_zgyro
  Bias2 : Bias  Bias=1717
  Bias3 : Bias  Bias=241
  Bias4 : Bias  Bias=-68
  Bias5 : Bias  Bias=42
  Bias6 : Bias  Bias=imuOffset_xacc
  Bias7 : Bias  Bias=imuOffset_yacc
  Bias8 : Bias  Bias=imuOffset_zacc
  Bias9 : Bias  Bias=imuOffset_xgyro
  Data Type Conversion{,1..3} (4 alike) : DataTypeConversion  OutDataTypeStr=int16  ConvertRealWorld=Stored Integer (SI)
  Demux{1..4} (4 alike) : Demux  Outputs=3
  Gain{1..4} (4 alike) : Gain  Gain=-1  RndMeth=Simplest  SaturateOnIntegerOverflow=on  OutDataTypeStr=Inherit: Same as input
  Mux{,1..3} (4 alike) : Mux  Inputs=3
  Scale rate Accel : DataTypeConversion  OutDataTypeStr=fixdt(1,16,4/65536,0)  ConvertRealWorld=Stored Integer (SI)
  Scale rate gyro : DataTypeConversion  OutDataTypeStr=fixdt(1,16,1000*pi/180/65536,0)  ConvertRealWorld=Stored Integer (SI)
  Gxyz : Outport
  Axyz : Outport  Port=2
  T : Outport  Port=3
  Axyz RAW : Outport  Port=4
  Gxyz RAW : Outport  Port=5
  wires:
  Data Type Conversion1/1 -> Demux2/1
  Bias3/1 -> Gain1/1
  Bias5/1 -> Gain2/1
  Demux2/1 -> Bias3/1  "U3 CH5"
  Demux1/2 -> Bias1/1  "U3 CH2"
  Demux2/2 -> Bias4/1  "U3 CH6"
  Demux1/3 -> Bias2/1  "U3 CH3"
  Demux1/1 -> Bias/1  "U3 CH1"
  "BUS SPI Read MPU 6050 Axyz, T°, Gxyz (100 Hz)"/1 -> Data Type Conversion3/1, Data Type Conversion/1  "U1 CH8"
  Demux2/3 -> Bias5/1  "U3 CH7"
  Data Type Conversion/1 -> Demux1/1
  Gain1/1 -> Mux1/1  "U3 CH5"
  Bias2/1 -> Gain4/1  "U3 CH3"
  "BUS SPI Read MPU 6050 Axyz, T°, Gxyz (100 Hz)"/2 -> T/1  "U3 CH4"
  Bias/1 -> Gain3/1  "U3 CH1"
  Mux/1 -> Scale rate Accel/1
  Gain2/1 -> Mux1/3  "U3 CH7"
  Bias1/1 -> Mux/2  "U3 CH2"
  Bias4/1 -> Mux1/2  "U3 CH6"
  Mux1/1 -> Scale rate gyro/1
  Scale rate gyro/1 -> Gxyz/1
  Scale rate Accel/1 -> Axyz/1
  Gain3/1 -> Mux/1
  Gain4/1 -> Mux/3
  Demux3/2 -> Bias7/1  "U3 CH2"
  Demux3/3 -> Bias8/1  "U3 CH3"
  Demux3/1 -> Bias6/1  "U3 CH1"
  Bias8/1 -> Mux2/3  "U3 CH3"
  Bias6/1 -> Mux2/1  "U3 CH1"
  Mux2/1 -> Axyz RAW/1
  Bias7/1 -> Mux2/2  "U3 CH2"
  "BUS SPI Read MPU 6050 Axyz, T°, Gxyz (100 Hz)"/3 -> Data Type Conversion1/1, Data Type Conversion2/1
  Demux4/1 -> Bias9/1  "U3 CH5"
  Demux4/2 -> Bias10/1  "U3 CH6"
  Demux4/3 -> Bias11/1  "U3 CH7"
  Bias9/1 -> Mux3/1  "U3 CH5"
  Bias11/1 -> Mux3/3  "U3 CH7"
  Bias10/1 -> Mux3/2  "U3 CH6"
  Mux3/1 -> Gxyz RAW/1
  Data Type Conversion2/1 -> Demux4/1
  Data Type Conversion3/1 -> Demux3/1

== system AUAV_V3_TestSensors/IMU_Mag_Driver/Disable path through in HIL Subsystem1 ==
  In1 : Inport
  In2 : Inport  Port=2
  In3 : Inport  Port=3
  In4 : Inport  Port=4
  In5 : Inport  Port=5
  In6 : Inport  Port=6
  In7 : Inport  Port=7
  In8 : Inport  Port=8
  In9 : Inport  Port=9
  In10 : Inport  Port=10
  Enable : EnablePort
  Update MPU_T1 : DataStoreWrite  DialogController=Simulink.DDGSource  DataStoreName=MPU_T  DataStoreElements=MPU_T
  Update Raw IMU DATA1 : DataStoreWrite  DialogController=Simulink.DDGSource  DataStoreName=mlRawImuData  DataStoreElements=mlRawImuData.xacc#mlRawImuData.yacc#mlRawImuData.zacc#mlRawImuData.xgyro#mlRawImuData.ygyro#mlRawImuData.zgyro#mlRawImuData.xmag#mlRawImuData.ymag#mlRawImuData.zmag
  wires:
  In1/1 -> Update Raw IMU DATA1/1
  In2/1 -> Update Raw IMU DATA1/2
  In3/1 -> Update Raw IMU DATA1/3
  In4/1 -> Update Raw IMU DATA1/4
  In5/1 -> Update Raw IMU DATA1/5
  In6/1 -> Update Raw IMU DATA1/6
  In7/1 -> Update Raw IMU DATA1/7
  In8/1 -> Update Raw IMU DATA1/8
  In9/1 -> Update Raw IMU DATA1/9
  In10/1 -> Update MPU_T1/1

== system AUAV_V3_TestSensors/IMU_Mag_Driver/Subsystem1 ==
  Hi : Inport
  Low : Inport  Port=2
  Bitwise Operator : simulink/Logic and Bit Operations/Bitwise Operator  logicop=OR  UseBitMask=off  NumInputPorts=2  BitMask=bin2dec('11011001')  BitMaskRealWorld=Stored Integer
  Data Type Conversion1 : DataTypeConversion  OutDataTypeStr=uint16  ConvertRealWorld=Stored Integer (SI)
  Data Type Conversion2 : DataTypeConversion  OutDataTypeStr=int16  ConvertRealWorld=Stored Integer (SI)
  Data Type Conversion3 : DataTypeConversion  OutDataTypeStr=uint16  ConvertRealWorld=Stored Integer (SI)
  Shift Arithmetic : ArithShift  BitShiftNumber=8
  Out1 : Outport
  wires:
  Hi/1 -> Data Type Conversion1/1
  Bitwise Operator/1 -> Data Type Conversion2/1
  Data Type Conversion2/1 -> Out1/1
  Data Type Conversion1/1 -> Shift Arithmetic/1
  Shift Arithmetic/1 -> Bitwise Operator/1
  Low/1 -> Data Type Conversion3/1
  Data Type Conversion3/1 -> Bitwise Operator/2

== system AUAV_V3_TestSensors/IMU_Mag_Driver/Subsystem10 ==
  Hi : Inport
  Low : Inport  Port=2
  Bitwise Operator : simulink/Logic and Bit Operations/Bitwise Operator  logicop=OR  UseBitMask=off  NumInputPorts=2  BitMask=bin2dec('11011001')  BitMaskRealWorld=Stored Integer
  Data Type Conversion1 : DataTypeConversion  OutDataTypeStr=uint16  ConvertRealWorld=Stored Integer (SI)
  Data Type Conversion2 : DataTypeConversion  OutDataTypeStr=int16  ConvertRealWorld=Stored Integer (SI)
  Data Type Conversion3 : DataTypeConversion  OutDataTypeStr=uint16  ConvertRealWorld=Stored Integer (SI)
  Shift Arithmetic : ArithShift  BitShiftNumber=8
  Out1 : Outport
  wires:
  Hi/1 -> Data Type Conversion1/1
  Bitwise Operator/1 -> Data Type Conversion2/1
  Data Type Conversion2/1 -> Out1/1
  Data Type Conversion1/1 -> Shift Arithmetic/1
  Shift Arithmetic/1 -> Bitwise Operator/1
  Low/1 -> Data Type Conversion3/1
  Data Type Conversion3/1 -> Bitwise Operator/2

== system AUAV_V3_TestSensors/IMU_Mag_Driver/Subsystem2 ==
  Hi : Inport
  Low : Inport  Port=2
  Bitwise Operator : simulink/Logic and Bit Operations/Bitwise Operator  logicop=OR  UseBitMask=off  NumInputPorts=2  BitMask=bin2dec('11011001')  BitMaskRealWorld=Stored Integer
  Data Type Conversion1 : DataTypeConversion  OutDataTypeStr=uint16  ConvertRealWorld=Stored Integer (SI)
  Data Type Conversion2 : DataTypeConversion  OutDataTypeStr=int16  ConvertRealWorld=Stored Integer (SI)
  Data Type Conversion3 : DataTypeConversion  OutDataTypeStr=uint16  ConvertRealWorld=Stored Integer (SI)
  Shift Arithmetic : ArithShift  BitShiftNumber=8
  Out1 : Outport
  wires:
  Hi/1 -> Data Type Conversion1/1
  Bitwise Operator/1 -> Data Type Conversion2/1
  Data Type Conversion2/1 -> Out1/1
  Data Type Conversion1/1 -> Shift Arithmetic/1
  Shift Arithmetic/1 -> Bitwise Operator/1
  Low/1 -> Data Type Conversion3/1
  Data Type Conversion3/1 -> Bitwise Operator/2

== system AUAV_V3_TestSensors/IMU_Mag_Driver/Subsystem3 ==
  Hi : Inport
  Low : Inport  Port=2
  Bitwise Operator : simulink/Logic and Bit Operations/Bitwise Operator  logicop=OR  UseBitMask=off  NumInputPorts=2  BitMask=bin2dec('11011001')  BitMaskRealWorld=Stored Integer
  Data Type Conversion1 : DataTypeConversion  OutDataTypeStr=uint16  ConvertRealWorld=Stored Integer (SI)
  Data Type Conversion2 : DataTypeConversion  OutDataTypeStr=int16  ConvertRealWorld=Stored Integer (SI)
  Data Type Conversion3 : DataTypeConversion  OutDataTypeStr=uint16  ConvertRealWorld=Stored Integer (SI)
  Shift Arithmetic : ArithShift  BitShiftNumber=8
  Out1 : Outport
  wires:
  Data Type Conversion3/1 -> Bitwise Operator/2
  Low/1 -> Data Type Conversion3/1
  Shift Arithmetic/1 -> Bitwise Operator/1
  Data Type Conversion1/1 -> Shift Arithmetic/1
  Data Type Conversion2/1 -> Out1/1
  Bitwise Operator/1 -> Data Type Conversion2/1
  Hi/1 -> Data Type Conversion1/1

== system AUAV_V3_TestSensors/IMU_Mag_Driver/Subsystem8 ==
  Hi : Inport
  Low : Inport  Port=2
  Bitwise Operator : simulink/Logic and Bit Operations/Bitwise Operator  logicop=OR  UseBitMask=off  NumInputPorts=2  BitMask=bin2dec('11011001')  BitMaskRealWorld=Stored Integer
  Data Type Conversion1 : DataTypeConversion  OutDataTypeStr=uint16  ConvertRealWorld=Stored Integer (SI)
  Data Type Conversion2 : DataTypeConversion  OutDataTypeStr=int16  ConvertRealWorld=Stored Integer (SI)
  Data Type Conversion3 : DataTypeConversion  OutDataTypeStr=uint16  ConvertRealWorld=Stored Integer (SI)
  Shift Arithmetic : ArithShift  BitShiftNumber=8
  Out1 : Outport
  wires:
  Hi/1 -> Data Type Conversion1/1
  Bitwise Operator/1 -> Data Type Conversion2/1
  Data Type Conversion2/1 -> Out1/1
  Data Type Conversion1/1 -> Shift Arithmetic/1
  Shift Arithmetic/1 -> Bitwise Operator/1
  Low/1 -> Data Type Conversion3/1
  Data Type Conversion3/1 -> Bitwise Operator/2

== system AUAV_V3_TestSensors/IMU_Mag_Driver/Subsystem9 ==
  Hi : Inport
  Low : Inport  Port=2
  Bitwise Operator : simulink/Logic and Bit Operations/Bitwise Operator  logicop=OR  UseBitMask=off  NumInputPorts=2  BitMask=bin2dec('11011001')  BitMaskRealWorld=Stored Integer
  Data Type Conversion1 : DataTypeConversion  OutDataTypeStr=uint16  ConvertRealWorld=Stored Integer (SI)
  Data Type Conversion2 : DataTypeConversion  OutDataTypeStr=int16  ConvertRealWorld=Stored Integer (SI)
  Data Type Conversion3 : DataTypeConversion  OutDataTypeStr=uint16  ConvertRealWorld=Stored Integer (SI)
  Shift Arithmetic : ArithShift  BitShiftNumber=8
  Out1 : Outport
  wires:
  Data Type Conversion3/1 -> Bitwise Operator/2
  Low/1 -> Data Type Conversion3/1
  Shift Arithmetic/1 -> Bitwise Operator/1
  Data Type Conversion1/1 -> Shift Arithmetic/1
  Data Type Conversion2/1 -> Out1/1
  Bitwise Operator/1 -> Data Type Conversion2/1
  Hi/1 -> Data Type Conversion1/1

== system AUAV_V3_TestSensors/Inner Loop// Navigation/Compute psi_dot_m ==
  r_m : Inport
  phi_m : Inport  Port=2
  q_m : Inport  Port=3
  Product : Product  SampleTime=apSampleTime  RndMeth=Zero
  Product1 : Product  SampleTime=apSampleTime  RndMeth=Zero
  Protect NaNs : Subsystem
  Subtract : Sum  Inputs=2
  dsPIC_cos : Subsystem  AncestorBlock=SLUGS_Library/dsPIC_cos
  dsPIC_sin : Subsystem  AncestorBlock=SLUGS_Library/dsPIC_sin
  psi_dot_m : Outport
  wires:
  q_m/1 -> Product1/1
  Subtract/1 -> Protect NaNs/1(In1)
  phi_m/1 -> dsPIC_sin/1(x), dsPIC_cos/1(u)
  r_m/1 -> Product/1
  Product1/1 -> Subtract/2
  Product/1 -> Subtract/1
  dsPIC_sin/1(sin(x)) -> Product1/2
  dsPIC_cos/1(cos(u)) -> Product/2
  Protect NaNs/1(Out1) -> psi_dot_m/1

== system AUAV_V3_TestSensors/Inner Loop// Navigation/L1 Output Feedback Controller With Projection Operator ==
  psi_dot_m : Inport
  m : Inport  Port=2
  omega : Inport  Port=3
  gamma : Inport  Port=4
  psi_dot_c : Inport  Port=5
  Enable : EnablePort  StatesWhenEnabling=reset  ShowOutputPort=on
  Constant : Constant  Value=2  OutDataTypeStr=single
  Constant1 : Constant  OutDataTypeStr=single
  Control Law : Subsystem
      mask Display:
      | droots([],'-a','a')
      | port_label('input',1,'a')
      | port_label('input',2,'u')
      | port_label('output',1,'y')
  Gain : Gain  Gain=-1  OutDataTypeStr=Inherit: Same as input
  Integer Delay : Delay  DelayLength=1  InputProcessing=Inherited  SampleTime=.01
  Integer Delay1 : Delay  DelayLength=1  InputProcessing=Inherited  SampleTime=.01
  Logical Operator : Logic  Operator=NOT  AllPortsSameDT=off  OutDataTypeStr=uint(8)
  Projection : Product  OutDataTypeStr=single  SampleTime=apSampleTime  RndMeth=Zero
  Projection Operator : Subsystem
  Protect NaNs : Subsystem
  Protect NaNs2 : Subsystem
  Psi Dot Limit : Saturate  UpperLimit=1  LowerLimit=-1  SampleTime=apSampleTime
  State Predictor : Subsystem
      mask Display:
      | droots([],'-a','a')
      | port_label('input',1,'a')
      | port_label('input',2,'u')
      | port_label('output',1,'y')
  Sum2 : Sum  Inputs=|++  OutDataTypeStr=single  SampleTime=apSampleTime
  Sum3 : Sum  Inputs=-+|  OutDataTypeStr=single  SampleTime=apSampleTime
  Sum4 : Sum  Inputs=+-|  OutDataTypeStr=single  SampleTime=apSampleTime
  Trapezoidal Integrator : Subsystem  AncestorBlock=SLUGS_Library/Control Blocks/PID Controller w//Anti-Windup/Trapezoidal Integrator  mask{T=apSampleTime, upperLimit=2, lowerLimit=-2}
      mask prompts: T "Sample Time"; upperLimit "Upper Saturation"; lowerLimit "Lower Saturation"
  psi_dot_ad : Outport
  wires:
  Integer Delay/1 -> Sum4/1  "psi_dot_c"
  State Predictor/1(y) -> Sum3/2
  Gain/1 -> Projection Operator/4(y)
  m/1 -> State Predictor/1(a)
  Sum2/1 -> Protect NaNs2/1(In1)
  psi_dot_m/1 -> Protect NaNs/1(In1)  "psi_dot_m"
  Sum3/1 -> Gain/1  "psi_dot_tilde"
  gamma/1 -> Projection/1  "adaptation gain"
  Projection/1 -> Trapezoidal Integrator/1(x)
  psi_dot_c/1 -> Integer Delay/1  "psi_dot_c"
  omega/1 -> Control Law/1(a)
  Control Law/1(y) -> Sum4/2  "sigma_hat_fil"
  Sum4/1 -> Psi Dot Limit/1  "psi_ad"
  Projection Operator/1("Proj(the, y)") -> Projection/2  "Proj"
  Constant/1 -> Projection Operator/1(Theta Max)
  Constant1/1 -> Projection Operator/2(Eps 0)
  Integer Delay1/1 -> Sum2/2, Projection Operator/3(Theta)
  Enable/1 -> Logical Operator/1
  Logical Operator/1 -> Trapezoidal Integrator/2(Reset)
  Trapezoidal Integrator/1(Int(x)) -> Control Law/2(u), Integer Delay1/1  "sigma_hat"
  Protect NaNs2/1(Out1) -> State Predictor/2(u)
  Protect NaNs/1(Out1) -> Sum3/1
  Psi Dot Limit/1 -> psi_dot_ad/1, Sum2/1

== system AUAV_V3_TestSensors/Inner Loop// Navigation/Lateral Channel Encaps [updated 4.28.16] ==
  r_m : Inport
  Manual? : Inport  Port=2
  Yaw Damp PID Gains : Inport  Port=3
  dR Trim : Inport  Port=4
  psi_dot_c_noNav : Inport  Port=5
  U_m : Inport  Port=6
  phi_m : Inport  Port=7
  Roll PID Gains : Inport  Port=8
  dA Trim : Inport  Port=9
  nav_phi_c : Inport  Port=10
  psi_dot_ad : Inport  Port=11  SampleTime=apSampleTime
  L1OnOff : Inport  Port=12
  Enable SS Comp : Inport  Port=13
  Ayb : Inport  Port=14
  dR Mix? : Inport  Port=15
  dR Mix gain : Inport  Port=16
  isPassthrough : Inport  Port=17
  Lateral Channel : Subsystem  AncestorBlock=SLUGS_Library/Control Blocks/Lateral Channel
  U_m1 : InportShadow  Port=6
  mlNavigation : DataStoreWrite  DialogController=Simulink.DDGSource  DataStoreName=mlNavigation  DataStoreElements=mlNavigation.psiDot_c#mlNavigation.phi_c#mlNavigation.ay_body
  psi_dot_c Select logic1 : Subsystem  AncestorBlock=SLUGS_Library/Control Blocks/psi_dot_c Select logic
  dA : Outport
  dR : Outport  Port=2
  phi_c : Outport  Port=3
  psi_dot_c_4_L1 : Outport  Port=4
  wires:
  Lateral Channel/4(psiDot) -> mlNavigation/1
  Lateral Channel/5(rHp) -> mlNavigation/3
  dR Trim/1 -> Lateral Channel/4(dR Trim)
  phi_m/1 -> Lateral Channel/7(phi_m)
  r_m/1 -> Lateral Channel/1(r_m)
  Lateral Channel/1(dA) -> dA/1
  Roll PID Gains/1 -> Lateral Channel/8(Roll PID Gains)
  dA Trim/1 -> Lateral Channel/9(dA Trim)
  Enable SS Comp/1 -> Lateral Channel/10(Enable SS Comp)
  Manual?/1 -> Lateral Channel/2(Manual?)
  Ayb/1 -> Lateral Channel/11(Ayb)
  dR Mix gain/1 -> Lateral Channel/13(dR Mix gain)
  Lateral Channel/2(dR) -> dR/1
  Yaw Damp PID Gains/1 -> Lateral Channel/3(Yaw Damp PID Gains)
  dR Mix?/1 -> Lateral Channel/12(dR Mix?)
  Lateral Channel/3(phi_c) -> mlNavigation/2, phi_c/1
  U_m/1 -> Lateral Channel/6(U_m)
  nav_phi_c/1 -> psi_dot_c Select logic1/5(nav_phi_c)
  U_m1/1 -> psi_dot_c Select logic1/6(U_m)
  psi_dot_ad/1 -> psi_dot_c Select logic1/1(psi_dot_ad)
  L1OnOff/1 -> psi_dot_c Select logic1/2(L1OnOff)
  psi_dot_c_noNav/1 -> psi_dot_c Select logic1/3(psi_dot_c_noNav)
  [psi_dot_c] -> Lateral Channel/5(psi_dot_c)
  psi_dot_c Select logic1/1(psi_dot_c) -> [psi_dot_c]
  psi_dot_c Select logic1/2(psi_dot_c_4_L1) -> psi_dot_c_4_L1/1
  isPassthrough/1 -> psi_dot_c Select logic1/4(IsPassThrough)

== system AUAV_V3_TestSensors/Inner Loop// Navigation/Longitudinal Channel Encaps [updated 4.28.16] ==
  U_c : Inport
  dyn P : Inport  Port=2
  U_hold PID Gains : Inport  Port=3
  dT_trim : Inport  Port=4
  h_c : Inport  Port=5
  h_m : Inport  Port=6
  he2th PI Gains : Inport  Port=7
  Roll to Height FF : Inport  Port=8
  theta_m : Inport  Port=9
  th2dE PID Gains : Inport  Port=10
  dE_trim : Inport  Port=11
  Manual? : Inport  Port=12
  phi_m : Inport  Port=13
  dt FF Gain : Inport  Port=14
  Constant3 : Constant  Value=[100 100 100]  OutDataTypeStr=single
  Longitudinal Channel : Subsystem  AncestorBlock=SLUGS_Library/Control Blocks/Longitudinal Channel
  mlNavigation : DataStoreWrite  DialogController=Simulink.DDGSource  DataStoreName=mlNavigation  DataStoreElements=mlNavigation.u_m#mlNavigation.theta_c#mlNavigation.h_c
  dE : Outport
  dT : Outport  Port=2
  theta_C : Outport  Port=3
  h_c_in : Outport  Port=4
  U_m : Outport  Port=5
  wires:
  U_c/1 -> Longitudinal Channel/1(U_c)
  dyn P/1 -> Longitudinal Channel/2(dyn P)
  U_hold PID Gains/1 -> Longitudinal Channel/3(U_hold PID Gains)
  dT_trim/1 -> Longitudinal Channel/4(dT_trim)
  h_m/1 -> Longitudinal Channel/6(h_m)
  theta_m/1 -> Longitudinal Channel/9(theta_m)
  dE_trim/1 -> Longitudinal Channel/11(dE_trim)
  Manual?/1 -> Longitudinal Channel/12(Manual?)
  he2th PI Gains/1 -> Longitudinal Channel/7(he2th PI Gains)
  Roll to Height FF/1 -> Longitudinal Channel/8(Roll to Height FF)
  th2dE PID Gains/1 -> Longitudinal Channel/10(th2dE PID Gains)
  dt FF Gain/1 -> Longitudinal Channel/14(dt FF Gain)
  h_c/1 -> Longitudinal Channel/5(h_c)
  phi_m/1 -> Longitudinal Channel/13(phi_m)
  Longitudinal Channel/1(dE) -> dE/1  "U"
  Longitudinal Channel/2(dT) -> dT/1
  Longitudinal Channel/3(h_c_in) -> mlNavigation/3, h_c_in/1
  Longitudinal Channel/4(U_m) -> mlNavigation/1, U_m/1
  Longitudinal Channel/5(theta_C) -> mlNavigation/2, theta_C/1
  Constant3/1 -> Longitudinal Channel/15(GS Location)
